simulink model "sldemo_mdlref_dsm_bot"  (Simulink 7.6)
settings: Solver=FixedStepDiscrete  StartTime=0.0  StopTime=10.0  FixedStep=0.1  RelTol=1e-3
settings Model: Creator=The MathWorks Inc.  ExtModeAutoUpdateStatusClock=off
settings OptimizationCC: InlineParams=on  InitFltsAndDblsToZero=on
settings DebuggingCC: SaveWithParameterizedLinksMsg=none  MultiTaskCondExecSysMsg=none  SigSpecEnsureSampleTimeMsg=none  BusObjectLabelMismatch=error  RootOutportRequireBusObject=error  StrictBusMsg=ErrorOnBusTreatedAsVector
settings RTWCC: ProcessScript=grt_make_rtw_hook  IncludeERTFirstTime=on
settings CodeAppCC: MaxIdLength=100
settings GRTTargetCC: TargetFcnLib=ansi_tfl_tmw.mat

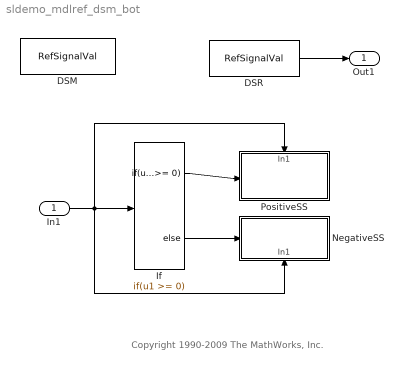
== system sldemo_mdlref_dsm_bot ==
  note: Copyright 1990-2009 The MathWorks, Inc.
  In1 : Inport  OutDataTypeStr=double  PortDimensions=1  SampleTime=0.1
  DSM : DataStoreMemory  DataStoreName=RefSignalVal  WriteAfterWriteMsg=warning
  DSR : DataStoreRead  DataStoreName=RefSignalVal  SampleTime=0.1
  If : If  IfExpression=u1 >= 0
  NegativeSS : Subsystem  TreatAsAtomicUnit=on
  PositiveSS : Subsystem  TreatAsAtomicUnit=on
  Out1 : Outport
  wires:
  DSR/1 -> Out1/1
  If/1 -> PositiveSS/Action
  If/2 -> NegativeSS/Action
  In1/1 -> If/1, PositiveSS/1(In1), NegativeSS/1(In1)

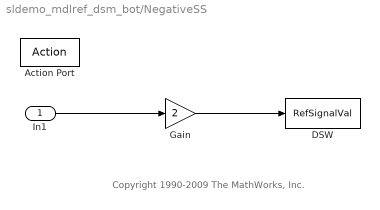
== system sldemo_mdlref_dsm_bot/NegativeSS ==
  note: Copyright 1990-2009 The MathWorks, Inc.
  In1 : Inport
  Action Port : ActionPort  ActionType=else
  DSW : DataStoreWrite  DataStoreName=RefSignalVal
  Gain : Gain  Gain=2
  wires:
  In1/1 -> Gain/1
  Gain/1 -> DSW/1

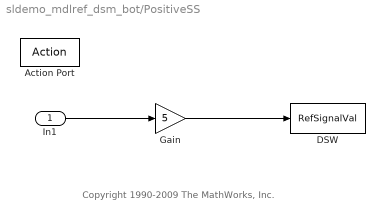
== system sldemo_mdlref_dsm_bot/PositiveSS ==
  note: Copyright 1990-2009 The MathWorks, Inc.
  In1 : Inport
  Action Port : ActionPort  ActionType=then
  DSW : DataStoreWrite  DataStoreName=RefSignalVal
  Gain : Gain  Gain=5
  wires:
  In1/1 -> Gain/1
  Gain/1 -> DSW/1
